simulink model "nid_thesis3"  (Simulink 8.1)
settings: Solver=FixedStepDiscrete  StartTime=0.0  StopTime=inf  RelTol=1e-3
libraries: nid_lib x2, visionsinks x1
settings Model: Creator=tchikama  LastModifiedBy=BeeLED
settings DataIOCC: SaveOutput=off
settings OptimizationCC: SimCompilerOptimization=On
settings HardwareCC: ProdIntDivRoundTo=Zero  ProdEndianess=LittleEndian  ProdHWDeviceType=Generic->32-bit x86 compatible
settings RTWCC: ProcessScript=grt_make_rtw_hook  RTWCompilerOptimization=On
settings CodeAppCC: MaxIdLength=95

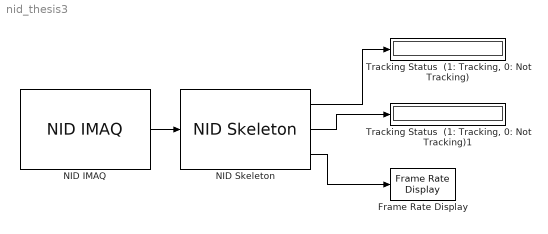
== system nid_thesis3 ==
  Frame Rate Display : visionsinks/Frame Rate Display  UpdateRate=10
  NID IMAQ : nid_lib/NID IMAQ  imaq_depth=off  imaq_motion=off  imaq_image=off  view_point=on  imaq_skeleton=on  imaq_ir=off  mirror_image=off  imaq_sample_time=1/30  res_fps=VGA (640x480): 30 FPS  needPsiPose=off  angle_input=off  angle=0  angle_read=off  near_mode=off  seated_mode=off  skeleton_smooth=[0.5 0.5 0.5 0.05 0.04]  infer_skeleton=on
  NID Skeleton : nid_lib/NID Skeleton  num_of_skeleton_tracking=1  conv_XYZ_RW=on  viewer=on
  "Tracking Status  (1: Tracking, 0: Not Tracking)" : Display
  "Tracking Status  (1: Tracking, 0: Not Tracking)1" : Display
  wires:
  NID IMAQ/1 -> NID Skeleton/1
  NID Skeleton/1 -> "Tracking Status  (1: Tracking, 0: Not Tracking)"/1
  NID Skeleton/3 -> Frame Rate Display/1
  NID Skeleton/2 -> "Tracking Status  (1: Tracking, 0: Not Tracking)1"/1
